simulink model "saildrone"  (R2022a)
settings: Solver=FixedStepAuto  StartTime=0.0  StopTime=10.0  RelTol=1e-3  EnableMultiTasking=on
undefined symbols (not defined in the file): dev, Main, pwm_output0
libraries: px4lib x2, simulink x1, etargetslib x1, px4Sensorslib x1
settings Model: ExtModeTrigDuration=10  Creator=kavin  LastModifiedBy=kavin
settings SolverCC: PositivePriorityOrder=on
settings OptimizationCC: EnhancedBackFolding=on  PassReuseOutputArgsAs=Individual arguments  ZeroExternalMemoryAtStartup=off  ZeroInternalMemoryAtStartup=off  MaxStackSize=64  OptimizeBlockOrder=speed  DifferentSizesBufferReuse=on  OptimizationCustomize=off  EfficientTunableParamExpr=on
settings DebuggingCC: ParameterTunabilityLossMsg=error
settings HardwareCC: ProdBitPerPointer=32  ProdBitPerSizeT=32  ProdBitPerPtrDiffT=32  ProdLargestAtomicInteger=Long  ProdLargestAtomicFloat=Double  ProdWordSize=32  ProdLongLongMode=on  ProdHWDeviceType=ARM Compatible->ARM Cortex
settings SFSimCC: MATLABDynamicMemAlloc=off  SimTargetLang=C++
settings RTWCC: SystemTargetFile=ert.tlc  HardwareBoard=PX4 Pixhawk 4  TLCOptions="-aInlineSetEventsForThisBaseRateFcn=TLC_FALSE -aSuppressMultiTaskScheduler=TLC_FALSE  -aRateBasedStepFcn=0"  TemplateMakefile=ert_default_tmf  Toolchain=GNU Tools for PX4 Autopilots  TargetLang=C++
settings CodeAppCC: ForceParamTrailComments=on  IgnoreCustomStorageClasses=off  OperatorAnnotations=on  SimulinkDataObjDesc=on  SFDataObjDesc=on  InsertBlockDesc=on
settings ERTTargetCC: ExtModeTransport=3  ExtModeStaticAlloc=on  ExtModeStaticAllocSize=1024  ExtModeMexFile=ext_xcp  ExtModeIntrfLevel=Level2 - Open

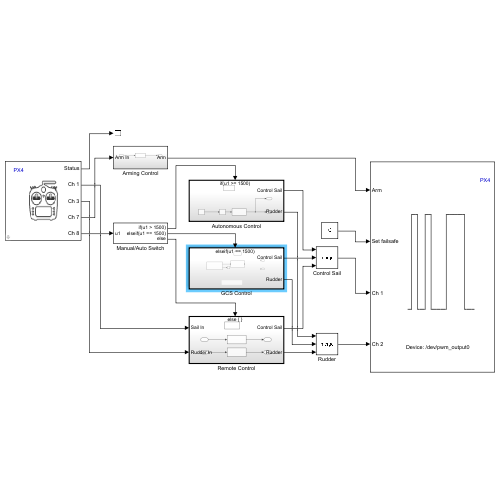
[thumbnail: Simulink's stored preview of the top-level diagram]
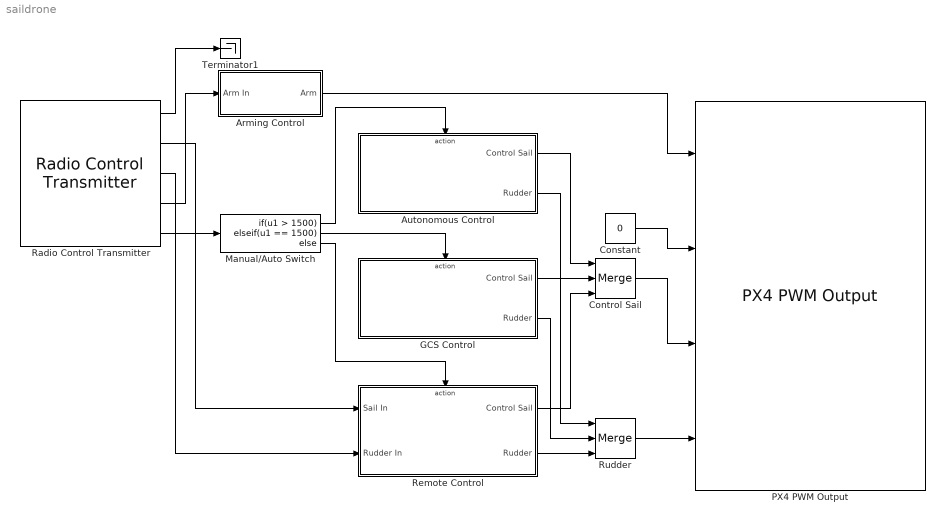
== system saildrone ==
  Arming Control : Subsystem
  Autonomous Control : Subsystem  TreatAsAtomicUnit=on
  Constant : Constant  Value=0  OutDataTypeStr=boolean
  Control Sail : Merge  Inputs=3
  GCS Control : Subsystem  TreatAsAtomicUnit=on
  Manual/Auto Switch : If  IfExpression=u1 > 1500  ElseIfExpressions=u1 == 1500
  PX4 PWM Output : px4lib/PX4 PWM Output  pwmDevice=Main (/dev/pwm_output0)  pwmChannel1_=on  pwmChannel2_=on  pwmChannel3_=off  pwmChannel4_=off  pwmChannel5_=off  pwmChannel6_=off  pwmChannel7_=off  pwmChannel8_=off  forceTerminateFailsafe=off  outputErrorStatus=off
      settings: SourceProductBaseCode=PX4AUTOPILOTS
  Radio Control Transmitter : px4Sensorslib/Radio Control Transmitter  channel1=on  channel2=off  channel3=on  channel4=off  channel5=off  channel6=off  channel7=on  channel8=on  channel_count=off  rssi=off  rc_input_source=off  timestamp_last_signal=off  time_stamp=off  sampleTime=1/250  BlockingMode=off  BlockTimeout=5
      settings: SourceProductBaseCode=PX4AUTOPILOTS
  Remote Control : Subsystem  TreatAsAtomicUnit=on
  Rudder : Merge  Inputs=3
  Terminator1 : Terminator
  wires:
  GCS Control/1(Control Sail) -> Control Sail/2
  GCS Control/2(Rudder) -> Rudder/2
  Manual/Auto Switch/1 -> Autonomous Control/Action
  Arming Control/1(Arm) -> PX4 PWM Output/1
  Manual/Auto Switch/2 -> GCS Control/Action
  Radio Control Transmitter/5 -> Manual/Auto Switch/1
  Radio Control Transmitter/4 -> Arming Control/1(Arm In)
  Radio Control Transmitter/3 -> Remote Control/2(Rudder In)
  Rudder/1 -> PX4 PWM Output/4
  Radio Control Transmitter/1 -> Terminator1/1
  Radio Control Transmitter/2 -> Remote Control/1(Sail In)
  Remote Control/2(Rudder) -> Rudder/3
  Autonomous Control/2(Rudder) -> Rudder/1
  Control Sail/1 -> PX4 PWM Output/3
  Remote Control/1(Control Sail) -> Control Sail/3
  Autonomous Control/1(Control Sail) -> Control Sail/1
  Manual/Auto Switch/3 -> Remote Control/Action
  Constant/1 -> PX4 PWM Output/2

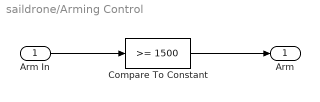
== system saildrone/Arming Control ==
  Arm In : Inport
  Compare To Constant : simulink/Logic and Bit Operations/Compare To Constant  relop=>=  const=1500  OutDataTypeStr=boolean
  Arm : Outport
  wires:
  Arm In/1 -> Compare To Constant/1
  Compare To Constant/1 -> Arm/1

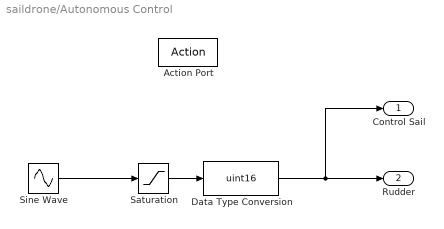
== system saildrone/Autonomous Control ==
  Action Port : ActionPort  ActionPortLabel=if(u1 >= 1500)
  Data Type Conversion : DataTypeConversion  OutDataTypeStr=uint16  SaturateOnIntegerOverflow=off  RndMeth=Floor
  Saturation : Saturate  UpperLimit=2000  LowerLimit=1000
  Sine Wave : Sin  Amplitude=400  Bias=1500  Frequency=3  SampleTime=0.004
  Control Sail : Outport
  Rudder : Outport  Port=2
  wires:
  Sine Wave/1 -> Saturation/1
  Saturation/1 -> Data Type Conversion/1
  Data Type Conversion/1 -> Control Sail/1, Rudder/1

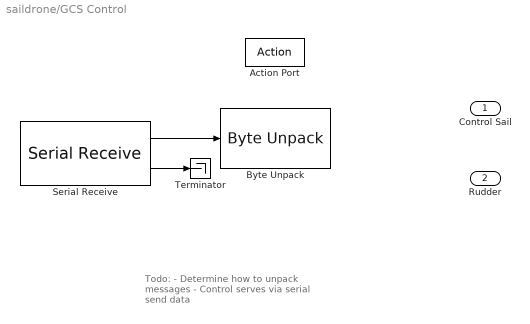
== system saildrone/GCS Control ==
  note: Todo:
      | - Determine how to unpack messages
      | - Control serves via serial send data
  Action Port : ActionPort  ActionPortLabel=elseif(u1 == 1500)
  Byte Unpack : etargetslib/Byte Unpack  dimensions={[4]}  datatypes={'uint16'}  byteAlign=1
  Serial Receive : px4lib/Serial Receive  SCIModule=/dev/ttyS1  DataType=uint16  DataLength=5  OutputStatus=on  SampleTime=0.1  BlockingMode=off  PartialData=off  Timeout=5
      settings: SourceProductBaseCode=PX4AUTOPILOTS
  Terminator : Terminator
  Control Sail : Outport
  Rudder : Outport  Port=2
  wires:
  Serial Receive/2 -> Terminator/1
  Serial Receive/1 -> Byte Unpack/1

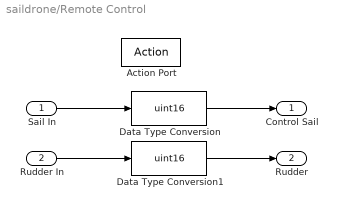
== system saildrone/Remote Control ==
  Sail In : Inport
  Rudder In : Inport  Port=2
  Action Port : ActionPort  ActionPortLabel=else
  Data Type Conversion : DataTypeConversion  OutDataTypeStr=uint16  SaturateOnIntegerOverflow=off  RndMeth=Floor
  Data Type Conversion1 : DataTypeConversion  OutDataTypeStr=uint16  SaturateOnIntegerOverflow=off  RndMeth=Floor
  Control Sail : Outport
  Rudder : Outport  Port=2
  wires:
  Sail In/1 -> Data Type Conversion/1
  Rudder In/1 -> Data Type Conversion1/1
  Data Type Conversion/1 -> Control Sail/1
  Data Type Conversion1/1 -> Rudder/1
